simulink model "Model0611"  (R2014a)
settings: Solver=ode45  SolverMode=SingleTasking  StartTime=0.0  StopTime=3000  RelTol=1e-5
settings Model: CovMetricSettings=dwe  CovHtmlReporting=off  covSaveCumulativeToWorkspaceVar=off  CovSaveSingleToWorkspaceVar=off  CovExternalEMLEnable=on  CovSFcnEnable=on  Creator=22875  LastModifiedBy=22875
settings DataIOCC: LimitDataPoints=off
settings DebuggingCC: MergeDetectMultiDrivingBlocksExec=error  SolverPrmCheckMsg=none  FrameProcessingCompatibilityMsg=error  SFUnexpectedBacktrackingDiag=error  SFNoUnconditionalDefaultTransitionDiag=error
settings HardwareCC: ProdBitPerPointer=64  ProdLargestAtomicFloat=Float  ProdIntDivRoundTo=Zero  ProdEndianess=LittleEndian  ProdHWDeviceType=Specified
settings ModelReferenceCC: PropagateSignalLabelsOutOfModel=on
settings GRTTargetCC: TargetLangStandard=C99 (ISO)  GeneratePreprocessorConditionals=Use local settings

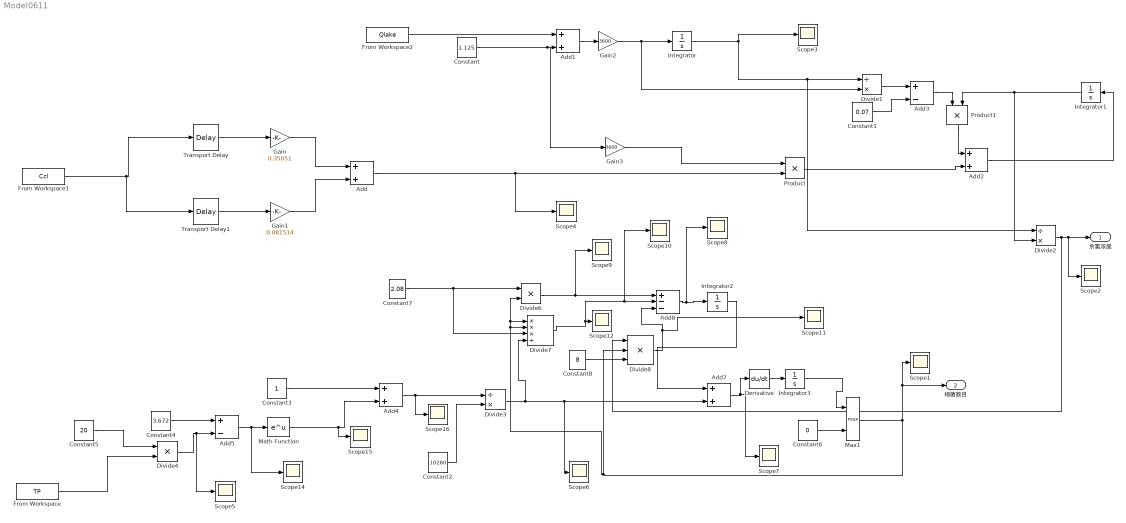
== system Model0611 ==
  Add{,1..2,4,7} (5 alike) : Sum
  Add3 : Sum  Inputs=+-
  Add5 : Sum  Inputs=+-
  Add8 : Sum  Inputs=+--
  Constant : Constant  Value=1.125
  Constant1 : Constant  Value=0.07
  Constant2 : Constant  Value=10280
  Constant3 : Constant
  Constant4 : Constant  Value=3.672
  Constant5 : Constant  Value=20
  Constant6 : Constant  Value=0
  Constant7 : Constant  Value=2.08
  Constant8 : Constant  Value=8
  Derivative : Derivative
  Divide1 : Product  Inputs=/*
  Divide2 : Product  Inputs=/*
  Divide3 : Product  Inputs=/*
  Divide4 : Product  Inputs=**
  Divide6 : Product  Inputs=**
  Divide7 : Product  Inputs=***/
  Divide8 : Product  Inputs=***
  From Workspace : FromWorkspace  VariableName=TP  SampleTime=0
  From Workspace1 : FromWorkspace  VariableName=Ccl  SampleTime=0
  From Workspace2 : FromWorkspace  VariableName=Qlake  SampleTime=0
  Gain : Gain  Gain=0.35051
  Gain1 : Gain  Gain=0.081514
  Gain2 : Gain  Gain=3600
  Gain3 : Gain  Gain=3600
  Integrator : Integrator  InitialCondition=540000
  Integrator1 : Integrator
  Integrator2 : Integrator  LimitOutput=on  UpperSaturationLimit=80000  LowerSaturationLimit=-80000  IgnoreLimit=on
  Integrator3 : Integrator  InitialCondition=2500  UpperSaturationLimit=15000  LowerSaturationLimit=0
  Math Function : Math  SaturateOnIntegerOverflow=on
  Max1 : MinMax  Function=max  Inputs=2
  Product : Product
  Product1 : Product
  Scope{1..12,14..16} (15 alike) : Scope
      Scope1 settings: TimeRange=auto  MaxDataPoints=5000  SaveToWorkspace=off  YMin=456.45102  YMax=4283.74893  SampleTime=-1
      Scope10 settings: TimeRange=auto  MaxDataPoints=5000  SaveToWorkspace=off  SaveName=ScopeData2  YMin=-2480.20214  YMax=24578.82477  SampleTime=-1
      Scope11 settings: TimeRange=auto  MaxDataPoints=5000  SaveToWorkspace=off  SaveName=ScopeData3  YMin=-963.10304  YMax=8667.92739  SampleTime=-1
      Scope12 settings: TimeRange=auto  MaxDataPoints=5000  SaveToWorkspace=off  SaveName=ScopeData4  YMin=-2480.20214  YMax=24578.82477  SampleTime=-1
      Scope14 settings: TimeRange=auto  MaxDataPoints=5000  SaveToWorkspace=off  SaveName=ScopeData6  YMin=-13.32191  YMax=-4.91098  SampleTime=-1
      Scope15 settings: TimeRange=auto  MaxDataPoints=5000  SaveToWorkspace=off  SaveName=ScopeData7  YMin=-0.00039  YMax=0.00357  SampleTime=-1
      Scope16 settings: TimeRange=auto  MaxDataPoints=5000  SaveToWorkspace=off  SaveName=ScopeData8  YMin=0.99643  YMax=1.00039  SampleTime=-1
      Scope2 settings: TimeRange=auto  MaxDataPoints=5000  SaveToWorkspace=off  SaveName=ScopeData  YMin=-0.01208  YMax=0.10876  SampleTime=-1
      Scope3 settings: TimeRange=auto  MaxDataPoints=5000  SaveToWorkspace=off  SaveName=ScopeData2  YMin=-2812367.0568  YMax=912485.22853  SampleTime=-1
      Scope4 settings: TimeRange=auto  MaxDataPoints=5000  SaveToWorkspace=off  SaveName=ScopeData3  YMin=-0.49684  YMax=4.47156  SampleTime=-1
      Scope5 settings: TimeRange=auto  MaxDataPoints=5000  SaveToWorkspace=off  SaveName=ScopeData4  YMin=8.58298  YMax=16.99391  SampleTime=-1
      Scope6 settings: TimeRange=auto  MaxDataPoints=5000  SaveToWorkspace=off  SaveName=ScopeData5  YMin=493.72906  YMax=5165.01153  SampleTime=-1
      Scope7 settings: TimeRange=auto  MaxDataPoints=5000  SaveToWorkspace=off  SaveName=ScopeData6  YMin=-1000.00001  YMax=8999.99999  SampleTime=-1
      Scope8 settings: TimeRange=auto  MaxDataPoints=5000  SaveToWorkspace=off  SaveName=ScopeData7  YMin=-13942772319.50502  YMax=1549196927.16682  SampleTime=-1
      Scope9 settings: TimeRange=auto  MaxDataPoints=5000  SaveToWorkspace=off  YMin=-111.59101  YMax=11584.29412  SampleTime=-1
  Transport Delay : TransportDelay  DelayTime=5.5
  Transport Delay1 : TransportDelay  DelayTime=2.92
  "余氯浓度 " : Outport
  细菌数目 : Outport  Port=2
  wires:
  From Workspace1/1 -> Transport Delay1/1, Transport Delay/1
  Transport Delay1/1 -> Gain1/1
  Transport Delay/1 -> Gain/1
  Gain/1 -> Add/1
  Gain1/1 -> Add/2
  Add/1 -> Product/2, Scope4/1
  Add1/1 -> Gain2/1
  Integrator/1 -> Scope3/1, Divide2/1, Divide1/1
  From Workspace2/1 -> Add1/1
  Constant/1 -> Gain3/1, Add1/2
  Product/1 -> Add2/2
  Divide1/1 -> Add3/1
  Constant1/1 -> Add3/2
  Add2/1 -> Integrator1/1
  Integrator1/1 -> Divide2/2, Product1/2
  Product1/1 -> Add2/1
  Add3/1 -> Product1/1
  Divide2/1 -> Divide8/1, Scope2/1, "余氯浓度 "/1
  Gain2/1 -> Divide1/2, Integrator/1
  Gain3/1 -> Product/1
  Constant2/1 -> Divide3/2
  Add4/1 -> Scope16/1, Divide3/1
  Constant3/1 -> Add4/1
  Math Function/1 -> Scope15/1, Add4/2
  Add5/1 -> Scope14/1, Math Function/1
  Constant4/1 -> Add5/1
  Constant5/1 -> Divide4/1
  From Workspace/1 -> Divide4/2
  Divide3/1 -> Divide7/4, Scope6/1, Add7/2
  Add7/1 -> Scope7/1, Derivative/1
  Constant7/1 -> Divide7/3, Divide6/1
  Divide6/1 -> Scope9/1, Add8/1
  Divide7/1 -> Scope12/1, Scope10/1, Add8/2
  Constant8/1 -> Divide8/3
  Divide8/1 -> Scope11/1, Add8/3
  Add8/1 -> Integrator2/1, Scope8/1
  Derivative/1 -> Integrator3/1
  Integrator3/1 -> Max1/1
  Divide4/1 -> Scope5/1, Add5/2
  Integrator2/1 -> Add7/1
  Constant6/1 -> Max1/2
  Max1/1 -> Scope1/1, 细菌数目/1, Divide7/2, Divide6/2, Divide7/1, Divide8/2
